simulink model "Atmos_VarConst"  (R2016b)
settings: Solver=VariableStepAuto  StartTime=0.0  StopTime=10.0  RelTol=1e-3
undefined symbols (not defined in the file or in its folder): Env
settings Model: Creator=rega0051  LastModifiedBy=rega0051
settings DataIOCC: SaveOutput=off  SignalLogging=off  DSMLogging=off  SaveTime=off

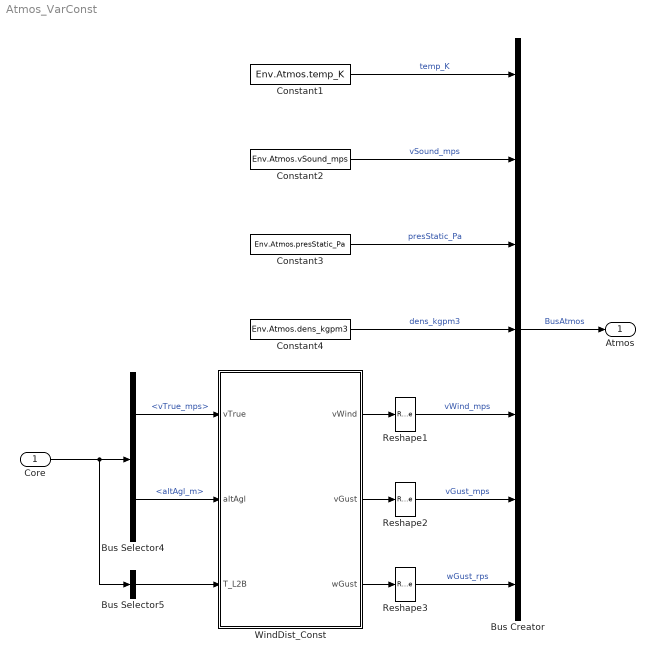
== system Atmos_VarConst ==
  Core : Inport  OutDataTypeStr=Bus: BusCore
      settings: AttributesFormatString=%<OutDataTypeStr>
  Bus Creator : BusCreator  Inputs=7  OutDataTypeStr=Bus: BusAtmos
      settings: AttributesFormatString=%<OutDataTypeStr>
  Bus Selector4 : BusSelector  OutputSignals=BusAux.BusFlow.vTrue_mps,BusAux.BusNav.altAgl_m
  Bus Selector5 : BusSelector  OutputSignals=BusEom.T_L2B  OutputAsBus=on
  Constant1 : Constant  Value=Env.Atmos.temp_K
      settings: AttributesFormatString=%<Value>
  Constant2 : Constant  Value=Env.Atmos.vSound_mps
      settings: AttributesFormatString=%<Value>
  Constant3 : Constant  Value=Env.Atmos.presStatic_Pa
      settings: AttributesFormatString=%<Value>
  Constant4 : Constant  Value=Env.Atmos.dens_kgpm3
      settings: AttributesFormatString=%<Value>
  Reshape1 : Reshape  OutputDimensionality=Column vector (2-D)  OutputDimensions=[3,1]
  Reshape2 : Reshape  OutputDimensionality=Column vector (2-D)  OutputDimensions=[3,1]
  Reshape3 : Reshape  OutputDimensionality=Column vector (2-D)  OutputDimensions=[3,1]
  WindDist_Const : Subsystem
      settings: MinAlgLoopOccurrences=on
  Atmos : Outport  OutDataTypeStr=Bus: BusAtmos
      settings: AttributesFormatString=%<OutDataTypeStr>
  wires:
  Reshape3/1 -> Bus Creator/7  "wGust_rps"
  Reshape2/1 -> Bus Creator/6  "vGust_mps"
  Reshape1/1 -> Bus Creator/5  "vWind_mps"
  Bus Creator/1 -> Atmos/1  "BusAtmos"
  Core/1 -> Bus Selector5/1, Bus Selector4/1
  Constant1/1 -> Bus Creator/1  "temp_K"
  WindDist_Const/1(vWind) -> Reshape1/1
  WindDist_Const/3(wGust) -> Reshape3/1
  Constant2/1 -> Bus Creator/2  "vSound_mps"
  Constant3/1 -> Bus Creator/3  "presStatic_Pa"
  WindDist_Const/2(vGust) -> Reshape2/1
  Constant4/1 -> Bus Creator/4  "dens_kgpm3"
  Bus Selector4/1 -> WindDist_Const/1(vTrue)  "<vTrue_mps>"
  Bus Selector4/2 -> WindDist_Const/2(altAgl)  "<altAgl_m>"
  Bus Selector5/1 -> WindDist_Const/3(T_L2B)

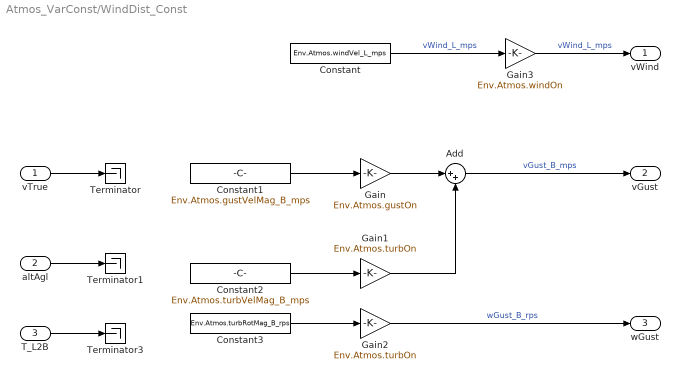
== system Atmos_VarConst/WindDist_Const ==
  vTrue : Inport
  altAgl : Inport  Port=2
  T_L2B : Inport  Port=3
  Add : Sum  Inputs=|++
  Constant : Constant  Value=Env.Atmos.windVel_L_mps
      settings: AttributesFormatString=%<Value>
  Constant1 : Constant  Value=Env.Atmos.gustVelMag_B_mps
      settings: AttributesFormatString=%<Value>
  Constant2 : Constant  Value=Env.Atmos.turbVelMag_B_mps
      settings: AttributesFormatString=%<Value>
  Constant3 : Constant  Value=Env.Atmos.turbRotMag_B_rps
      settings: AttributesFormatString=%<Value>
  Gain : Gain  Gain=Env.Atmos.gustOn
      settings: AttributesFormatString=%<Gain>
  Gain1 : Gain  Gain=Env.Atmos.turbOn
      settings: AttributesFormatString=%<Gain>
  Gain2 : Gain  Gain=Env.Atmos.turbOn
      settings: AttributesFormatString=%<Gain>
  Gain3 : Gain  Gain=Env.Atmos.windOn
      settings: AttributesFormatString=%<Gain>
  Terminator : Terminator
  Terminator1 : Terminator
  Terminator3 : Terminator
  vWind : Outport
  vGust : Outport  Port=2
  wGust : Outport  Port=3
  wires:
  Gain2/1 -> wGust/1  "wGust_B_rps"
  Add/1 -> vGust/1  "vGust_B_mps"
  altAgl/1 -> Terminator1/1
  T_L2B/1 -> Terminator3/1
  Constant3/1 -> Gain2/1
  Gain1/1 -> Add/2
  Gain/1 -> Add/1
  Gain3/1 -> vWind/1  "vWind_L_mps"
  Constant2/1 -> Gain1/1
  Constant1/1 -> Gain/1
  Constant/1 -> Gain3/1  "vWind_L_mps"
  vTrue/1 -> Terminator/1
